simulink subsystem "Plant_DMPC"  (R2023a)
settings: Solver=VariableStepAuto  StartTime=0.0  StopTime=10.0  RelTol=1e-3
settings Model: Creator=giaco  LastModifiedBy=giaco

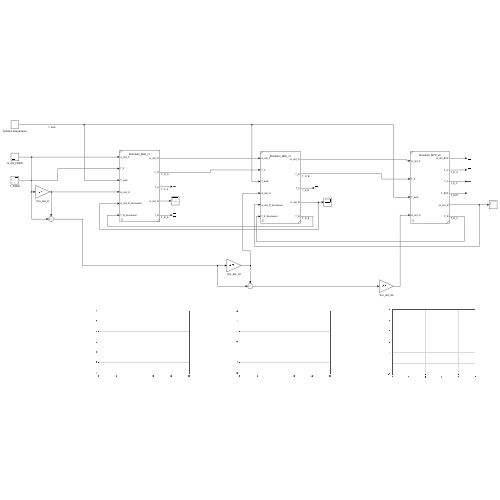
[thumbnail: Simulink's stored preview of the top-level diagram]
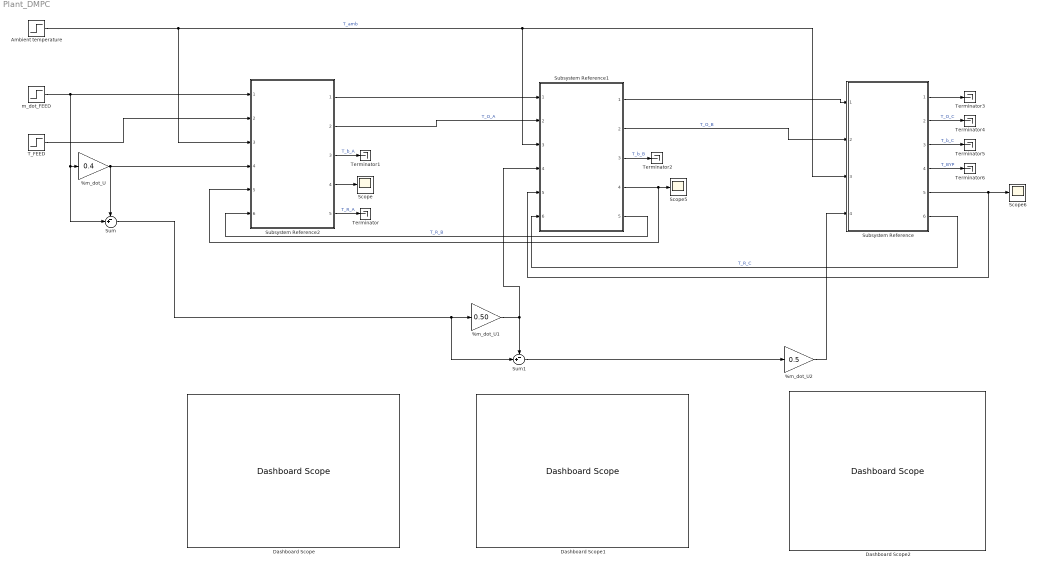
== system Plant_DMPC ==
  %m_dot_U : Gain  Gain=0.4
  %m_dot_U1 : Gain  Gain=0.50
  %m_dot_U2 : Gain  Gain=0.5
  Ambient temperature : Step  After=300  SampleTime=0
  Dashboard Scope : DashboardScope
  Dashboard Scope1 : DashboardScope
  Dashboard Scope2 : DashboardScope
  Scope : Scope
  Scope5 : Scope
  Scope6 : Scope
  Subsystem Reference : Subsystem  ReferencedSubsystem=Simulator_BYP_v0  rho=971  rho_air=971  c_p=4179  c_p_air=4179  pi=3.14151  L_F=40.5  D_F=0.4  h_F=1.5  D_S1=0.1  L_S1=5  h_S1=1.5  D_S2=0.025  L_S2=5000  h_S2=300  D_S3=0.1  L_S3=5  h_S3=1.5  D_R=0.4  L_R=40  h_R=1.5  C_b=100  A_b=500  h_b=1.5  D_BYP=0.1  L_BYP=3  h_BYP=1.5  T_F_0=273  T_S1_0=273  T_S2_0=273  T_S3_0=273  T_b_0=273  T_R_0=273
  Subsystem Reference1 : Subsystem  ReferencedSubsystem=Simulator_MID_v1  rho=971  rho_air=971  c_p=4179  c_p_air=4179  pi=3.14151  L_F=40.5  D_F=0.4  h_F=1.5  D_S1=0.1  L_S1=5  h_S1=1.5  D_S2=0.02  L_S2=50  h_S2=1.5  D_S3=0.1  L_S3=5  h_S3=1.5  D_R=0.4  L_R=40  h_R=1.5  C_b=300  A_b=500  h_b=1.5  T_F_0=273  T_S1_0=273  T_S2_0=273  T_S3_0=273  T_b_0=273  T_R_0=273
  Subsystem Reference2 : Subsystem  ReferencedSubsystem=Simulator_MID_v1  rho=971  rho_air=971  c_p=4179  c_p_air=4179  pi=3.14151  L_F=40.5  D_F=0.4  h_F=1.5  D_S1=0.1  L_S1=5  h_S1=1.5  D_S2=0.02  L_S2=50  h_S2=1.5  D_S3=0.1  L_S3=5  h_S3=1.5  D_R=0.4  L_R=40  h_R=1.5  C_b=300  A_b=500  h_b=1.5  T_F_0=273  T_S1_0=273  T_S2_0=273  T_S3_0=273  T_b_0=273  T_R_0=273
  Sum : Sum  Inputs=-+|
  Sum1 : Sum  Inputs=-+|
  T_FEED : Step  Time=0  After=350  SampleTime=0
  Terminator{,1..6} (7 alike) : Terminator
  m_dot_FEED : Step  Time=0  After=0.1  SampleTime=0
  wires:
  Subsystem Reference/3 -> Terminator5/1  "T_b_C"
  %m_dot_U/1 -> Subsystem Reference2/4, Sum/1
  Subsystem Reference/4 -> Terminator6/1  "T_BYP"
  Subsystem Reference1/2 -> Subsystem Reference/2  "T_O_B"
  Subsystem Reference/1 -> Terminator3/1
  Subsystem Reference1/3 -> Terminator2/1  "T_b_B"
  Subsystem Reference1/1 -> Subsystem Reference/1
  Sum1/1 -> %m_dot_U2/1
  Subsystem Reference2/1 -> Subsystem Reference1/1
  Subsystem Reference2/5 -> Terminator/1  "T_R_A"
  Ambient temperature/1 -> Subsystem Reference2/3, Subsystem Reference/3, Subsystem Reference1/3  "T_amb"
  Subsystem Reference/6 -> Subsystem Reference1/6  "T_R_C"
  %m_dot_U2/1 -> Subsystem Reference/4
  %m_dot_U1/1 -> Subsystem Reference1/4, Sum1/1
  Subsystem Reference1/4 -> Scope5/1, Subsystem Reference2/5
  Subsystem Reference1/5 -> Subsystem Reference2/6  "T_R_B"
  Subsystem Reference2/2 -> Subsystem Reference1/2  "T_O_A"
  Sum/1 -> Sum1/2, %m_dot_U1/1
  T_FEED/1 -> Subsystem Reference2/2
  Subsystem Reference/2 -> Terminator4/1  "T_O_C"
  m_dot_FEED/1 -> %m_dot_U/1, Sum/2, Subsystem Reference2/1
  Subsystem Reference2/4 -> Scope/1
  Subsystem Reference2/3 -> Terminator1/1  "T_b_A"
  Subsystem Reference/5 -> Scope6/1, Subsystem Reference1/5
